simulink model "EEPROM_M24C04_Demo"  (R2024b)
settings: Solver=FixedStepAuto  StartTime=0.0  StopTime=2.0  FixedStep=0.1  RelTol=1e-3
settings Model: Creator=Shreyas  LastModifiedBy=Shreyas
settings SFSimCC: SimCustomSourceCode="#include \"m24c04.c\""  SimCustomHeaderCode="#include \"m24c04.h\""
settings RTWCC: CustomSourceCode="#include \"m24c04.c\""  CustomHeaderCode="#include \"m24c04.h\""

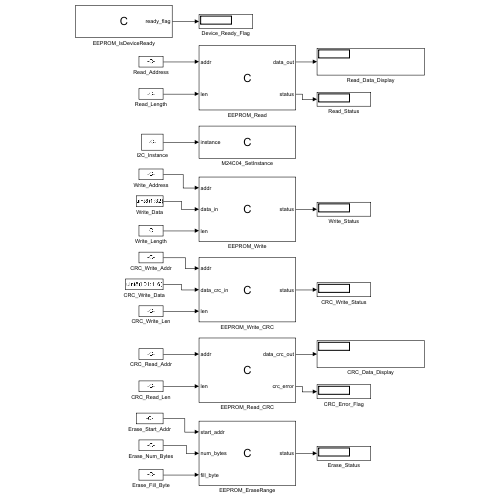
[thumbnail: Simulink's stored preview of the top-level diagram]
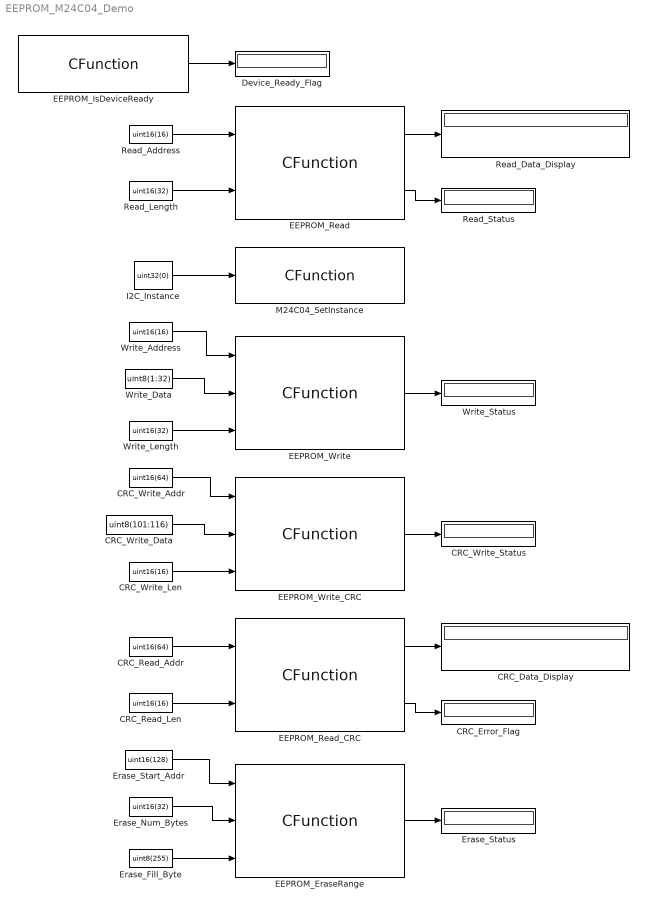
== system EEPROM_M24C04_Demo ==
  CRC_Data_Display : Display
  CRC_Error_Flag : Display
  CRC_Read_Addr : Constant  Value=uint16(64)  OutDataTypeStr=uint16
  CRC_Read_Len : Constant  Value=uint16(16)  OutDataTypeStr=uint16
  CRC_Write_Addr : Constant  Value=uint16(64)  OutDataTypeStr=uint16
  CRC_Write_Data : Constant  Value=uint8(101:116)  OutDataTypeStr=uint8
  CRC_Write_Len : Constant  Value=uint16(16)  OutDataTypeStr=uint16
  CRC_Write_Status : Display
  Device_Ready_Flag : Display
  EEPROM_EraseRange : CFunction  OutputCode=|  CodegenOutputCode=|  SimCustomHeaderFile=m24c04.h  SimCustomSourceFile=m24c04.c  CustomHeaderFile=m24c04.h  CustomSourceFile=m24c04.c  CustomCodeIsMultiInstantiable=on
      OutputCode=|
      | /* Blank EEPROM Range with pattern (e.g. 0xFF) */
      | status = M24C04_EraseRange(start_addr, num_bytes, fill_byte);
      CodegenOutputCode=|
      | /* Blank EEPROM Range with pattern (e.g. 0xFF) */
      | status = M24C04_EraseRange(start_addr, num_bytes, fill_byte);
  EEPROM_IsDeviceReady : CFunction  OutputCode=|  CodegenOutputCode=|  SimCustomHeaderFile=m24c04.h  SimCustomSourceFile=m24c04.c  CustomHeaderFile=m24c04.h  CustomSourceFile=m24c04.c  CustomCodeIsMultiInstantiable=on
      OutputCode=|
      | /* Acknowledge Polling: Query Chip Ready State after Write Cycle (t_W) */
      | ready_flag = (uint8_t)M24C04_IsDeviceReady();
      CodegenOutputCode=|
      | /* Acknowledge Polling: Query Chip Ready State after Write Cycle (t_W) */
      | ready_flag = (uint8_t)M24C04_IsDeviceReady();
  EEPROM_Read : CFunction  OutputCode=|  CodegenOutputCode=|  SimCustomHeaderFile=m24c04.h  SimCustomSourceFile=m24c04.c  CustomHeaderFile=m24c04.h  CustomSourceFile=m24c04.c  CustomCodeIsMultiInstantiable=on
      OutputCode=|
      | /* ST M24C04 Multi-Byte Sequential Read */
      | status = M24C04_ReadMulti(addr, data_out, len);
      CodegenOutputCode=|
      | /* ST M24C04 Multi-Byte Sequential Read */
      | status = M24C04_ReadMulti(addr, data_out, len);
  EEPROM_Read_CRC : CFunction  OutputCode=|  CodegenOutputCode=|  SimCustomHeaderFile=m24c04.h  SimCustomSourceFile=m24c04.c  CustomHeaderFile=m24c04.h  CustomSourceFile=m24c04.c  CustomCodeIsMultiInstantiable=on
      OutputCode=|
      | /* Safety Read: Verifies against stored SAE J1850 CRC-8 (0=Match, 4=Mismatch) */
      | crc_error = M24C04_ReadWithCRC(addr, data_crc_out, len);
      CodegenOutputCode=|
      | /* Safety Read: Verifies against stored SAE J1850 CRC-8 (0=Match, 4=Mismatch) */
      | crc_error = M24C04_ReadWithCRC(addr, data_crc_out, len);
  EEPROM_Write : CFunction  OutputCode=|  CodegenOutputCode=|  SimCustomHeaderFile=m24c04.h  SimCustomSourceFile=m24c04.c  CustomHeaderFile=m24c04.h  CustomSourceFile=m24c04.c  CustomCodeIsMultiInstantiable=on
      OutputCode=|
      | /* ST M24C04 Multi-Byte Safe Page Write */
      | status = M24C04_WriteMulti(addr, data_in, len);
      CodegenOutputCode=|
      | /* ST M24C04 Multi-Byte Safe Page Write */
      | status = M24C04_WriteMulti(addr, data_in, len);
  EEPROM_Write_CRC : CFunction  OutputCode=|  CodegenOutputCode=|  SimCustomHeaderFile=m24c04.h  SimCustomSourceFile=m24c04.c  CustomHeaderFile=m24c04.h  CustomSourceFile=m24c04.c  CustomCodeIsMultiInstantiable=on
      OutputCode=|
      | /* Safety Write: Appends Automotive SAE J1850 CRC-8 */
      | status = M24C04_WriteWithCRC(addr, data_crc_in, len);
      CodegenOutputCode=|
      | /* Safety Write: Appends Automotive SAE J1850 CRC-8 */
      | status = M24C04_WriteWithCRC(addr, data_crc_in, len);
  Erase_Fill_Byte : Constant  Value=uint8(255)  OutDataTypeStr=uint8
  Erase_Num_Bytes : Constant  Value=uint16(32)  OutDataTypeStr=uint16
  Erase_Start_Addr : Constant  Value=uint16(128)  OutDataTypeStr=uint16
  Erase_Status : Display
  I2C_Instance : Constant  Value=uint32(0)  OutDataTypeStr=uint32
  M24C04_SetInstance : CFunction  OutputCode=|  CodegenOutputCode=|  SimCustomHeaderFile=m24c04.h  SimCustomSourceFile=m24c04.c  CustomHeaderFile=m24c04.h  CustomSourceFile=m24c04.c  CustomCodeIsMultiInstantiable=on
      OutputCode=|
      | /* Set LPI2C Hardware Instance (0 = LPI2C0, 1 = LPI2C1) */
      | M24C04_SetI2CInstance(instance);
      CodegenOutputCode=|
      | /* Set LPI2C Hardware Instance (0 = LPI2C0, 1 = LPI2C1) */
      | M24C04_SetI2CInstance(instance);
  Read_Address : Constant  Value=uint16(16)  OutDataTypeStr=uint16
  Read_Data_Display : Display
  Read_Length : Constant  Value=uint16(32)  OutDataTypeStr=uint16
  Read_Status : Display
  Write_Address : Constant  Value=uint16(16)  OutDataTypeStr=uint16
  Write_Data : Constant  Value=uint8(1:32)  OutDataTypeStr=uint8
  Write_Length : Constant  Value=uint16(32)  OutDataTypeStr=uint16
  Write_Status : Display
  wires:
  EEPROM_IsDeviceReady/1 -> Device_Ready_Flag/1
  Read_Address/1 -> EEPROM_Read/1
  Write_Length/1 -> EEPROM_Write/3
  Write_Data/1 -> EEPROM_Write/2
  Read_Length/1 -> EEPROM_Read/2
  Write_Address/1 -> EEPROM_Write/1
  I2C_Instance/1 -> M24C04_SetInstance/1
  CRC_Write_Addr/1 -> EEPROM_Write_CRC/1
  CRC_Write_Data/1 -> EEPROM_Write_CRC/2
  CRC_Write_Len/1 -> EEPROM_Write_CRC/3
  CRC_Read_Addr/1 -> EEPROM_Read_CRC/1
  CRC_Read_Len/1 -> EEPROM_Read_CRC/2
  Erase_Fill_Byte/1 -> EEPROM_EraseRange/3
  Erase_Start_Addr/1 -> EEPROM_EraseRange/1
  EEPROM_Write_CRC/1 -> CRC_Write_Status/1
  Erase_Num_Bytes/1 -> EEPROM_EraseRange/2
  EEPROM_Read/1 -> Read_Data_Display/1
  EEPROM_Read_CRC/1 -> CRC_Data_Display/1
  EEPROM_Read/2 -> Read_Status/1
  EEPROM_Write/1 -> Write_Status/1
  EEPROM_Read_CRC/2 -> CRC_Error_Flag/1
  EEPROM_EraseRange/1 -> Erase_Status/1
